simulink model "Use_Cases_N1_a"  (R2020b)
settings: Solver=ode3  StartTime=0.0  StopTime=inf  FixedStep=0.05  RelTol=1e-3
libraries: XBotBlockToolbox x2, simulink x1, Utilities x1

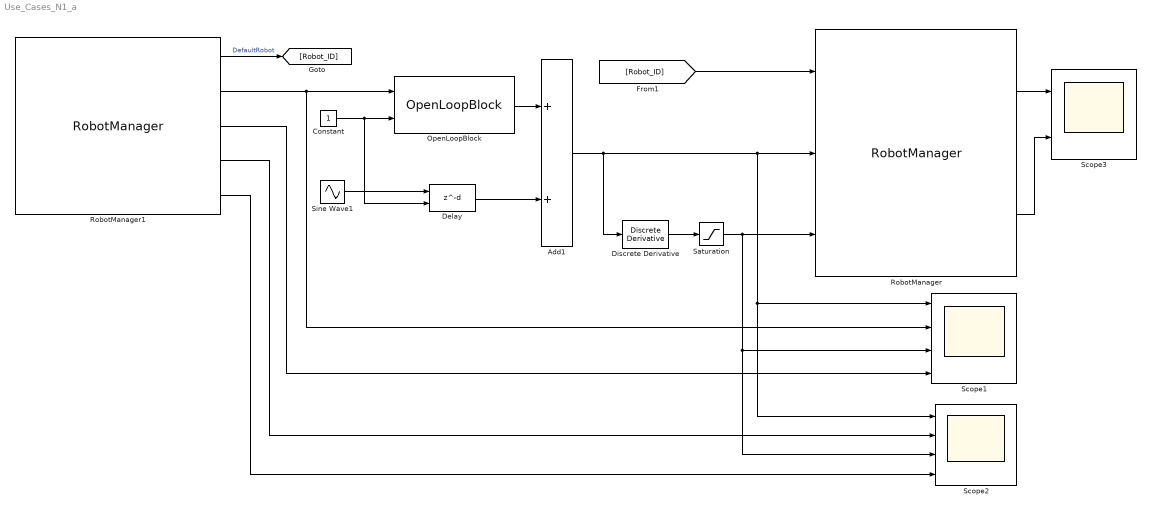
== system Use_Cases_N1_a ==
  Add1 : Sum
  Constant : Constant
  Delay : Delay  DelayLengthSource=Input port  DelayLength=1  InitialCondition=0
  Discrete Derivative : simulink/Discrete/Discrete Derivative  gainval=1.0  ICPrevScaledInput=0.0  OutMin=[]  OutMax=[]  OutDataType=fixdt(1, 16)  OutScaling=2^-10  DoSatur=off
  OpenLoopBlock : Utilities/OpenLoopBlock  SystemSampleTime=-1  VariantActivationTime=update diagram  Latency=0  AutoFrameSizeCalculation=off
  RobotManager : XBotBlockToolbox/RobotManager  RobotName=DefaultRobot  ModelName=DefaultRobot  UseExtRobot=On  SyncWithModel=Off  ReadingsList={}  MechanicalLimitsList={}  MechanicalLimitsCheck=On  MechanicalLimitsEnforce=On  SensorList={}  ReferencesList={ 'qJ_ref', 'qJdot_ref' }  OldRobotName=DefaultRobot
  RobotManager1 : XBotBlockToolbox/RobotManager  RobotName=DefaultRobot  ModelName=DefaultModel  UseExtRobot=Off  SyncWithModel=Off  ReadingsList={ 'qJ', 'qJdot', 'qJ_ref', 'qJdot_ref' }  MechanicalLimitsList={}  MechanicalLimitsCheck=Off  MechanicalLimitsEnforce=Off  SensorList={}  ReferencesList={}  OldRobotName=DefaultRobot
  Saturation : Saturate  UpperLimit=0.2  LowerLimit=-0.2
  Scope1 : Scope  NumInputPorts=4
  Scope2 : Scope  NumInputPorts=4
  Scope3 : Scope  NumInputPorts=2
  Sine Wave1 : Sin  Amplitude=0.2  SampleTime=0
  wires:
  RobotManager1/3 -> Scope1/4
  Add1/1 -> RobotManager/2, Scope1/1, Scope2/1, Discrete Derivative/1
  Sine Wave1/1 -> Delay/1
  Discrete Derivative/1 -> Saturation/1
  Saturation/1 -> RobotManager/3, Scope1/3, Scope2/3
  RobotManager1/2 -> Scope1/2, OpenLoopBlock/1
  OpenLoopBlock/1 -> Add1/1
  [Robot_ID] -> RobotManager/1
  RobotManager1/4 -> Scope2/2
  RobotManager1/5 -> Scope2/4
  RobotManager1/1 -> [Robot_ID]  "DefaultRobot"
  Constant/1 -> Delay/2, OpenLoopBlock/2
  RobotManager/1 -> Scope3/1
  RobotManager/2 -> Scope3/2
  Delay/1 -> Add1/2
